simulink subsystem "W9_Hydraulic_subsystem"  (R2020a)
settings: Solver=VariableStepAuto  StartTime=0.0  StopTime=10.0  RelTol=1e-3
undefined symbols (not defined in the file): WT_Params
libraries: Studio3_Actuator_library x3
settings Model: Creator=Emily  LastModifiedBy=Emily

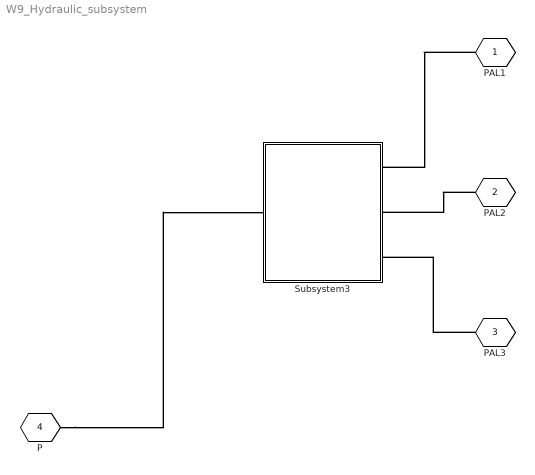
== system W9_Hydraulic_subsystem ==
  Subsystem3 : Subsystem
  PAL1 : PMIOPort  Tag=PMCPort  Side=Left
  PAL2 : PMIOPort  Tag=PMCPort  Port=2  Side=Left
  PAL3 : PMIOPort  Tag=PMCPort  Port=3  Side=Left
  P : PMIOPort  Tag=PMCPort  Port=4  Side=Left
  connections:
  PAL1/RConn1 -- Subsystem3/RConn1
  PAL2/RConn1 -- Subsystem3/RConn2
  PAL3/RConn1 -- Subsystem3/RConn3
  P/RConn1 -- Subsystem3/LConn1

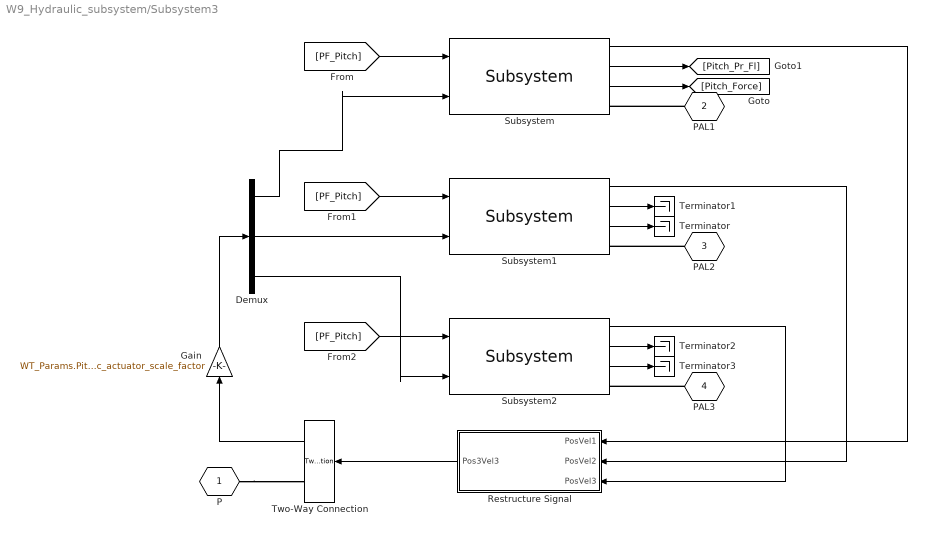
== system W9_Hydraulic_subsystem/Subsystem3 ==
  Demux : Demux  Outputs=3
  Gain : Gain  Gain=WT_Params.Pitch_Actuator.hydraulic_actuator_scale_factor
  Restructure Signal : Subsystem
  Subsystem : Studio3_Actuator_library/Subsystem  SystemSampleTime=-1  Latency=0  AutoFrameSizeCalculation=off
  Subsystem1 : Studio3_Actuator_library/Subsystem  SystemSampleTime=-1  Latency=0  AutoFrameSizeCalculation=off
  Subsystem2 : Studio3_Actuator_library/Subsystem  SystemSampleTime=-1  Latency=0  AutoFrameSizeCalculation=off
  Terminator{,1..3} (4 alike) : Terminator
  Two-Way Connection : TwoWayConnection
  P : PMIOPort  Tag=PMCPort  Side=Left
  PAL1 : PMIOPort  Tag=PMCPort  Port=2  Side=Right
  PAL2 : PMIOPort  Tag=PMCPort  Port=3  Side=Right
  PAL3 : PMIOPort  Tag=PMCPort  Port=4  Side=Right
  wires:
  Demux/3 -> Subsystem2/2
  Subsystem1/3 -> Terminator/1
  Restructure Signal/1(Pos3Vel3) -> Two-Way Connection/1
  Subsystem2/3 -> Terminator3/1
  [PF_Pitch] -> Subsystem2/1
  [PF_Pitch] -> Subsystem/1
  Demux/1 -> Subsystem/2
  [PF_Pitch] -> Subsystem1/1
  Subsystem1/2 -> Terminator1/1
  Subsystem2/2 -> Terminator2/1
  Two-Way Connection/1 -> Gain/1
  Demux/2 -> Subsystem1/2
  Subsystem/3 -> [Pitch_Force]
  Subsystem/2 -> [Pitch_Pr_Fl]
  Gain/1 -> Demux/1
  Subsystem/1 -> Restructure Signal/1(PosVel1)
  Subsystem1/1 -> Restructure Signal/2(PosVel2)
  Subsystem2/1 -> Restructure Signal/3(PosVel3)
  connections:
  P/RConn1 -- Two-Way Connection/RConn1
  PAL2/RConn1 -- Subsystem1/RConn1
  PAL1/RConn1 -- Subsystem/RConn1
  PAL3/RConn1 -- Subsystem2/RConn1

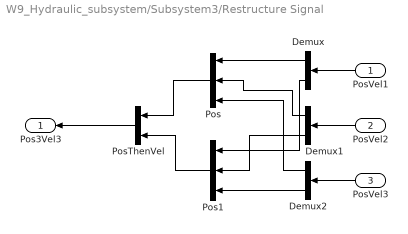
== system W9_Hydraulic_subsystem/Subsystem3/Restructure Signal ==
  PosVel1 : Inport
  PosVel2 : Inport  Port=2
  PosVel3 : Inport  Port=3
  Demux : Demux  Outputs=2
  Demux1 : Demux  Outputs=2
  Demux2 : Demux  Outputs=2
  Pos : Mux  Inputs=3
  Pos1 : Mux  Inputs=3
  PosThenVel : Mux  Inputs=2
  Pos3Vel3 : Outport
  wires:
  PosVel3/1 -> Demux2/1
  Pos/1 -> PosThenVel/1
  Demux/2 -> Pos1/1
  Demux1/2 -> Pos1/2
  Demux2/1 -> Pos/3
  Pos1/1 -> PosThenVel/2
  Demux/1 -> Pos/1
  PosVel1/1 -> Demux/1
  PosVel2/1 -> Demux1/1
  Demux2/2 -> Pos1/3
  PosThenVel/1 -> Pos3Vel3/1
  Demux1/1 -> Pos/2
